simulink model "sim_tutorial"  (Simulink 10.0)
settings: Solver=ode23tb  StartTime=0.0  StopTime=10  RelTol=1e-3  AbsTol=1e-5  EnableMultiTasking=on
undefined symbols (not defined in the file): a, bu, c, du, Rot
libraries: simulink3 x3
settings Model: Creator=bhisma  LastModifiedBy=bhisma  ExtModeTrigMode=oneshot  ExtModeArmWhenConnect=off
settings DataIOCC: SignalLoggingSaveFormat=ModelDataLogs
settings OptimizationCC: BlockReduction=off  BooleanDataType=off  LifeSpan=auto
settings DebuggingCC: SaveWithParameterizedLinksMsg=none  SignalResolutionControl=TryResolveAllWithWarning  MultiTaskDSMMsg=warning  MultiTaskCondExecSysMsg=none  SFUnexpectedBacktrackingDiag=error  SFNoUnconditionalDefaultTransitionDiag=error  SFExecutionAtInitializationDiag=warning  ArithmeticOperatorsInVariantConditions=error
settings HardwareCC: ProdBitPerPointer=64  ProdBitPerSizeT=64  ProdBitPerPtrDiffT=64  ProdLargestAtomicFloat=Float  ProdIntDivRoundTo=Zero  ProdEndianess=LittleEndian  ProdWordSize=64  ProdHWDeviceType=Intel->x86-64 (Windows64)  TargetUnknown=on
settings SFSimCC: SimUseLocalCustomCode=on  CustomCodeUndefinedFunction=FilterOut
settings RTWCC: RTWUseLocalCustomCode=on
settings CodeAppCC: StateflowObjectComments=off
settings GRTTargetCC: TargetLangStandard=C99 (ISO)
settings ConfigComp: CovMetricSettings=dwe  CovHtmlReporting=off  CovSaveCumulativeToWorkspaceVar=off  CovSaveSingleToWorkspaceVar=off

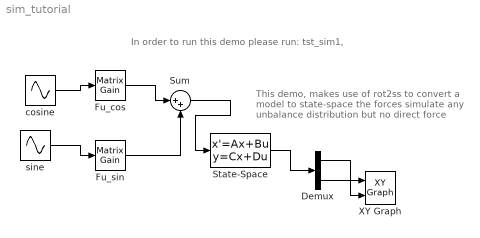
== system sim_tutorial ==
  note: In order to run this demo
      | please run:  tst_sim1,
  note: This demo, makes use of
      | rot2ss to convert a model to state-space
      | the forces simulate any unbalance distribution
      | but no direct force
  Demux : Demux  Outputs=2
  Fu_cos : simulink3/Math/Matrix Gain  K=Rot.Fu_cos
      settings: SourceProductName=Simulink  SourceProductBaseCode=SL
  Fu_sin : simulink3/Math/Matrix Gain  K=Rot.Fu_sin
      settings: SourceProductName=Simulink  SourceProductBaseCode=SL
  State-Space : StateSpace  A=a  B=bu  C=c  D=du  InitialCondition=0
  Sum : Sum  Inputs=|++  SaturateOnIntegerOverflow=on  InputSameDT=on  OutDataTypeStr=Inherit: Same as first input
  XY Graph : simulink3/Sinks/XY Graph  xmin=-2e-6  xmax=2e-6  ymin=-2e-6  ymax=2e-6  st=-1
      settings: SourceProductName=Simulink  SourceProductBaseCode=SL
  cosine : Sin  Frequency=Rot.W  Phase=pi/2  SampleTime=0
  sine : Sin  Frequency=Rot.W  SampleTime=0
  wires:
  cosine/1 -> Fu_cos/1
  sine/1 -> Fu_sin/1
  Sum/1 -> State-Space/1
  Fu_cos/1 -> Sum/1
  Fu_sin/1 -> Sum/2
  Demux/1 -> XY Graph/1
  Demux/2 -> XY Graph/2
  State-Space/1 -> Demux/1
